simulink model "Data_GeneratorDOF6"  (R2018b)
settings: Solver=FixedStepAuto  StartTime=0.0  StopTime=60  FixedStep=0.05  RelTol=1e-3
libraries: simulink_extras x1
settings Model: Creator=root  LastModifiedBy=root

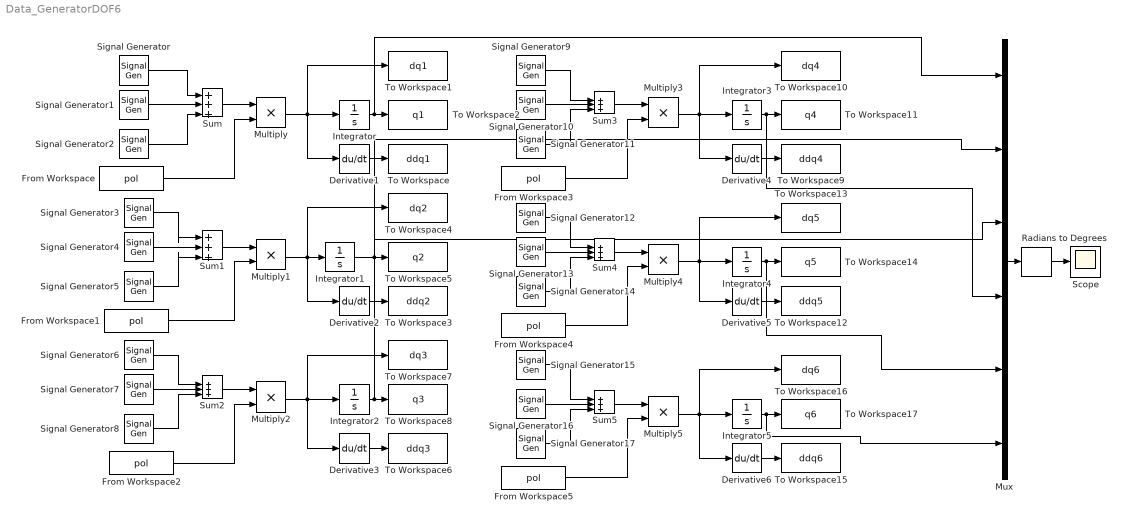
== system Data_GeneratorDOF6 ==
  Derivative{1..6} (6 alike) : Derivative
  From Workspace{,3..5} (4 alike) : FromWorkspace  VariableName=pol
  From Workspace1 : FromWorkspace  VariableName=pol  SampleTime=0
  From Workspace2 : FromWorkspace  VariableName=pol  SampleTime=0
  Integrator{,2,4..5} (4 alike) : Integrator
  Integrator1 : Integrator  InitialCondition=-pi/2
  Integrator3 : Integrator  InitialCondition=-pi/2
  Multiply{,1..5} (6 alike) : Product
  Mux : Mux  Inputs=6
  Radians to Degrees : simulink_extras/Transformations/Radians to Degrees
  Scope : Scope
  Signal Generator : SignalGenerator  Amplitude=0.12  Frequency=1.25  Units=rad/sec
  Signal Generator1 : SignalGenerator  Amplitude=0.12  Frequency=0.95  Units=rad/sec
  Signal Generator10 : SignalGenerator  Amplitude=-0.1  Units=rad/sec
  Signal Generator11 : SignalGenerator  Amplitude=-0.1  Frequency=0.4  Units=rad/sec
  Signal Generator12 : SignalGenerator  Amplitude=0.12  Units=rad/sec
  Signal Generator13 : SignalGenerator  Amplitude=0.12  Frequency=0.66  Units=rad/sec
  Signal Generator14 : SignalGenerator  Amplitude=0.12  Frequency=0.33  Units=rad/sec
  Signal Generator15 : SignalGenerator  Amplitude=0.3  Frequency=0.45  Units=rad/sec
  Signal Generator16 : SignalGenerator  Amplitude=0.3  Frequency=0.5  Units=rad/sec
  Signal Generator17 : SignalGenerator  Amplitude=0.3  Frequency=0.125  Units=rad/sec
  Signal Generator2 : SignalGenerator  Amplitude=-0.15  Units=rad/sec
  Signal Generator3 : SignalGenerator  Amplitude=0.1  Frequency=1.3  Units=rad/sec
  Signal Generator4 : SignalGenerator  Amplitude=0.1  Frequency=0.85  Units=rad/sec
  Signal Generator5 : SignalGenerator  Amplitude=-0.12  Frequency=0.25  Units=rad/sec
  Signal Generator6 : SignalGenerator  Amplitude=0.1  Frequency=2.5  Units=rad/sec
  Signal Generator7 : SignalGenerator  Amplitude=0.1  Frequency=2  Units=rad/sec
  Signal Generator8 : SignalGenerator  Amplitude=0.1  Frequency=0.85  Units=rad/sec
  Signal Generator9 : SignalGenerator  Amplitude=0.2  Frequency=0.4  Units=rad/sec
  Sum{,1..5} (6 alike) : Sum  Inputs=|+++
  To Workspace : ToWorkspace  VariableName=ddq1  SampleTime=-1
  To Workspace1 : ToWorkspace  VariableName=dq1  SampleTime=-1
  To Workspace10 : ToWorkspace  VariableName=dq4  SampleTime=-1
  To Workspace11 : ToWorkspace  VariableName=q4  SampleTime=-1
  To Workspace12 : ToWorkspace  VariableName=ddq5  SampleTime=-1
  To Workspace13 : ToWorkspace  VariableName=dq5  SampleTime=-1
  To Workspace14 : ToWorkspace  VariableName=q5  SampleTime=-1
  To Workspace15 : ToWorkspace  VariableName=ddq6  SampleTime=-1
  To Workspace16 : ToWorkspace  VariableName=dq6  SampleTime=-1
  To Workspace17 : ToWorkspace  VariableName=q6  SampleTime=-1
  To Workspace2 : ToWorkspace  VariableName=q1  SampleTime=-1
  To Workspace3 : ToWorkspace  VariableName=ddq2  SampleTime=-1
  To Workspace4 : ToWorkspace  VariableName=dq2  SampleTime=-1
  To Workspace5 : ToWorkspace  VariableName=q2  SampleTime=-1
  To Workspace6 : ToWorkspace  VariableName=ddq3  SampleTime=-1
  To Workspace7 : ToWorkspace  VariableName=dq3  SampleTime=-1
  To Workspace8 : ToWorkspace  VariableName=q3  SampleTime=-1
  To Workspace9 : ToWorkspace  VariableName=ddq4  SampleTime=-1
  wires:
  Signal Generator/1 -> Sum/1
  Signal Generator1/1 -> Sum/2
  Signal Generator2/1 -> Sum/3
  Integrator/1 -> Mux/1, To Workspace2/1
  Derivative1/1 -> To Workspace/1
  Derivative2/1 -> To Workspace3/1
  Signal Generator5/1 -> Sum1/3
  Signal Generator3/1 -> Sum1/1
  Signal Generator4/1 -> Sum1/2
  Integrator2/1 -> Mux/3, To Workspace8/1
  Derivative3/1 -> To Workspace6/1
  Signal Generator8/1 -> Sum2/3
  Signal Generator6/1 -> Sum2/1
  Signal Generator7/1 -> Sum2/2
  Integrator3/1 -> Mux/4, To Workspace11/1
  Derivative4/1 -> To Workspace9/1
  Signal Generator11/1 -> Sum3/3
  Signal Generator9/1 -> Sum3/1
  Signal Generator10/1 -> Sum3/2
  Integrator4/1 -> Mux/5, To Workspace14/1
  Derivative5/1 -> To Workspace12/1
  Signal Generator14/1 -> Sum4/3
  Signal Generator12/1 -> Sum4/1
  Signal Generator13/1 -> Sum4/2
  Integrator5/1 -> Mux/6, To Workspace17/1
  Derivative6/1 -> To Workspace15/1
  Signal Generator17/1 -> Sum5/3
  Signal Generator15/1 -> Sum5/1
  Signal Generator16/1 -> Sum5/2
  Multiply/1 -> Derivative1/1, To Workspace1/1, Integrator/1
  From Workspace/1 -> Multiply/2
  Sum/1 -> Multiply/1
  Multiply1/1 -> Integrator1/1, To Workspace4/1, Derivative2/1
  From Workspace1/1 -> Multiply1/2
  Sum1/1 -> Multiply1/1
  Sum2/1 -> Multiply2/1
  From Workspace2/1 -> Multiply2/2
  Multiply2/1 -> To Workspace7/1, Derivative3/1, Integrator2/1
  Sum3/1 -> Multiply3/1
  From Workspace3/1 -> Multiply3/2
  Multiply3/1 -> Integrator3/1, To Workspace10/1, Derivative4/1
  Sum4/1 -> Multiply4/1
  From Workspace4/1 -> Multiply4/2
  Multiply4/1 -> To Workspace13/1, Derivative5/1, Integrator4/1
  Sum5/1 -> Multiply5/1
  Multiply5/1 -> Derivative6/1, Integrator5/1, To Workspace16/1
  From Workspace5/1 -> Multiply5/2
  Integrator1/1 -> Mux/2, To Workspace5/1
  Mux/1 -> Radians to Degrees/1
  Radians to Degrees/1 -> Scope/1
